simulink model "Moteur_BF"  (R2018a)
settings: Solver=ode45  StartTime=0.0  StopTime=simTime  RelTol=1e-3
undefined symbols (not defined in the file): Kd_m, Ki_m, Km, Kp_m, targetAccel, targetSpeed, Tau_m
libraries: simulink x1
settings Model: Creator=chsira  LastModifiedBy=charl
settings SolverCC: MaxConsecutiveZCs=10000
settings DebuggingCC: MaxConsecutiveZCsMsg=none  LibraryContextMissingDiagnostic=warning
settings SFSimCC: SimUseLocalCustomCode=on
settings RTWCC: RTWUseLocalCustomCode=on

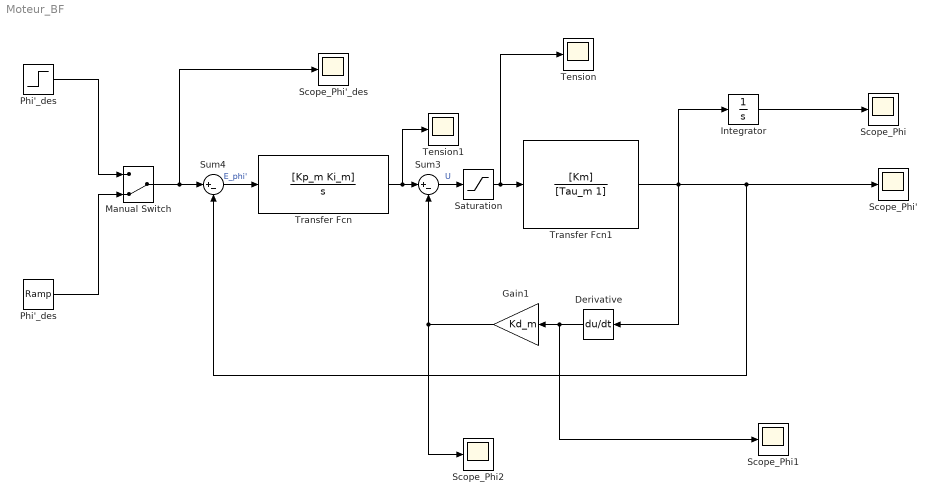
== system Moteur_BF ==
  Derivative : Derivative
  Gain1 : Gain  Gain=Kd_m
  Integrator : Integrator
  Manual Switch : ManualSwitch  CurrentSetting=0
  Phi'_des : simulink/Sources/Ramp  slope=targetAccel  start=0  InitialOutput=0
  "Phi'_des " : Step  Time=0  After=targetSpeed  SampleTime=0
  Saturation : Saturate  UpperLimit=6  LowerLimit=-6
  Scope_Phi : Scope
  Scope_Phi' : Scope
  Scope_Phi'_des : Scope
  Scope_Phi1 : Scope
  Scope_Phi2 : Scope
  Sum3 : Sum  Inputs=|+-
  Sum4 : Sum  Inputs=|+-
  Tension : Scope
  Tension1 : Scope
  Transfer Fcn : TransferFcn  Numerator=[Kp_m Ki_m]  Denominator=[1 0]
  Transfer Fcn1 : TransferFcn  Numerator=[Km]  Denominator=[Tau_m 1]
  wires:
  Sum3/1 -> Saturation/1  "U"
  Sum4/1 -> Transfer Fcn/1  "E_phi'"
  Transfer Fcn/1 -> Tension1/1, Sum3/1
  "Phi'_des "/1 -> Manual Switch/1
  Phi'_des/1 -> Manual Switch/2
  Derivative/1 -> Gain1/1, Scope_Phi1/1
  Transfer Fcn1/1 -> Integrator/1, Derivative/1, Scope_Phi'/1, Sum4/2
  Manual Switch/1 -> Scope_Phi'_des/1, Sum4/1
  Integrator/1 -> Scope_Phi/1
  Saturation/1 -> Transfer Fcn1/1, Tension/1
  Gain1/1 -> Scope_Phi2/1, Sum3/2
